simulink model "MavicProComplete"  (R2019a)
settings: Solver=VariableStepAuto  StartTime=0  StopTime=125  FixedStep=.01  RelTol=1e-3  EnableMultiTasking=on
InitFcn:
  | load('params/batteryModelSfun.mat');
  | load('params/DJI.mat');
  | load('params/DJIquadModel_X.mat');
  | load('params/motor.mat');
  | load('params/soc_ocv_new.mat');
model workspace (MAT data in the model file):
  Sig = Simulink.Signal
  Sig.DataType = 'auto'
  Sig.Dimensions = -1
  Sig.DimensionsMode = 'auto'
  Sig.Complexity = 'auto'
  Sig.SampleTime = -1
  Sig.SamplingMode = 'auto'
values from neighbouring files (symbols this model uses):
  P = block.ContStates.Data(1)    [quadcopterDynamicsSFunctionMod.m]
  Phi = block.ContStates.Data(4)    [quadcopterDynamicsSFunctionMod.m]
  Psi = block.ContStates.Data(6)    [quadcopterDynamicsSFunctionMod.m]
  Q = block.ContStates.Data(2)    [quadcopterDynamicsSFunctionMod.m]
  R = block.ContStates.Data(3)    [quadcopterDynamicsSFunctionMod.m]
  The = block.ContStates.Data(5)    [quadcopterDynamicsSFunctionMod.m]
  Z = block.ContStates.Data(12)    [quadcopterDynamicsSFunctionMod.m]
undefined symbols (not defined in the file or in its folder): Motor, quadModel
libraries: simulink x7
(part 1 of 2)
Description:
  | This is a configurable quadcopter simulation.
  | This Simulink model demonstates attitude control.
  | 
  | Additional quadcopter modeling and simulation materials available at:
  | github.com/dch33/Quad-Sim
  | 
  | Copyright (C) 2014 D. Hartman, K. Landis, S. Moreno, J. Kim, M. Mehrer
  | 
  | License:
  |     This program is free software: you can redistribute it and/or modify
  |     it under the terms of the GNU LESSER GENERAL PUBLIC LICENSE as published by
  |     the Free Software Foundation, either version 3 of the License, or
  |     (at your option) any later version.
  | 
  |     This program is distributed in the hope that it will be useful,
  |     but WITHOUT ANY WARRANTY; without even the implied warranty of
  |     MERCHANTABILITY or FITNESS FOR A PARTICULAR PURPOSE.  See the
  |     GNU General Public License for more details.
  | 
  |     You should have received a copy of the GNU LESSER GENERAL PUBLIC LICENSE
  |     along with this program.  If not, see <http://www.gnu.org/licenses/>.
settings Model: ModifiedComment=tdarrah -- Tue Jun 04 09:34:35 2019 -- Version 1.40  Creator=David Hartman  LastModifiedBy=tdarrah
settings Model: ModifiedHistory=|
  | tdarrah -- Tue Jun 04 09:34:35 2019 -- Version 1.40
  | 
  | tdarrah -- Tue Jun 04 05:29:55 2019 -- Version 1.39
  | 
  | tdarrah -- Mon Jun 03 18:31:35 2019 -- Version 1.38
  | closed the battery loop
  | 
  | tdarrah -- Mon Jun 03 18:20:30 2019 -- Version 1.37
  | added battery
  | 
  | 
  | tdarrah -- Mon Jun 03 17:58:08 2019 -- Version 1.36
  | incorporated our motors in model
  | 
  | 
  | Sahai Couso -- Fri May 10 11:35:12 2019 -- Version 1.35
  | 
  | Sahai Couso -- Fri May 10 10:41:34 2019 -- Version 1.34
  | 
  | Sahai Couso -- Fri May 10 10:40:52 2019 -- Version 1.33
  | 
  | Sahai Couso -- Fri May 10 10:30:50 2019 -- Version 1.32
  | 
  | Sahai Couso -- Fri May 10 10:24:25 2019 -- Version 1.31
  | 
  | Sahai Couso -- Wed May 08 22:16:35 2019 -- Version 1.30
  | 
  | Sahai Couso -- Wed May 08 22:15:23 2019 -- Version 1.29
  | 
  | Sahai Couso -- Wed May 08 22:14:58 2019 -- Version 1.28
  | 
  | Sahai Couso -- Wed May 08 22:04:36 2019 -- Version 1.27
  | 
  | Sahai Couso -- Wed May 08 22:04:16 2019 -- Version 1.26
  | 
  | Sahai Couso -- Wed May 08 21:57:14 2019 -- Version 1.25
  | 
  | Sahai Couso -- Wed May 08 21:54:04 2019 -- Version 1.24
  | 
  | Sahai Couso -- Wed May 08 21:53:17 2019 -- Version 1.23
  | 
  | Sahai Couso -- Wed May 08 21:48:07 2019 -- Version 1.22
  | 
  | Sahai Couso -- Wed May 08 21:35:53 2019 -- Version 1.21
  | 
  | Sahai Couso -- Wed May 08 21:28:21 2019 -- Version 1.19
  | 
  | Sahai Couso -- Wed May 08 21:28:21 2019 -- Version 1.19
  | 
  | Sahai Couso -- Wed May 08 21:25:30 2019 -- Version 1.18
  | 
  | Sahai Couso -- Wed May 08 21:23:06 2019 -- Version 1.17
  | 
  | Sahai Couso -- Wed May 08 13:57:34 2019 -- Version 1.16
  | 
  | Sahai Couso -- Wed May 08 00:58:43 2019 -- Version 1.15
  | 
  | Sahai Couso -- Wed May 08 00:58:03 2019 -- Version 1.14
  | 
  | Sahai Couso -- Tue May 07 23:55:58 2019 -- Version 1.13
  | 
  | Sahai Couso -- Tue May 07 23:08:00 2019 -- Version 1.12
  | 
  | Sahai Couso -- Tue May 07 23:06:52 2019 -- Version 1.11
  | 
  | Sahai Couso -- Tue May 07 22:57:09 2019 -- Version 1.10
  | 
  | Sahai Couso -- Tue May 07 22:48:57 2019 -- Version 1.9
  | 
  | Sahai Couso -- Tue May 07 21:40:08 2019 -- Version 1.8
  | 
  | Yves -- Tue Apr 04 13:12:37 2017 -- Version 1.7
  | 
  | Yves -- Tue Apr 04 13:10:33 2017 -- Version 1.6
  | 
  | davidhartman -- Fri Jun 06 23:19:51 2014 -- Version 1.5
  | 
  | 
  | davidhartman -- Fri Jun 06 22:53:10 2014 -- Version 1.3
settings SolverCC: AlgebraicLoopSolver=LineSearch  AutoInsertRateTranBlk=on
settings DataIOCC: SaveFormat=Array  SignalLogging=off  ReturnWorkspaceOutputs=off
settings OptimizationCC: DefaultParameterBehavior=Inlined  LifeSpan=inf
settings DebuggingCC: UnderspecifiedInitializationDetection=Classic  MergeDetectMultiDrivingBlocksExec=none  SolverPrmCheckMsg=warning  UniqueDataStoreMsg=warning  StateNameClashWarn=warning  PregeneratedLibrarySubsystemCodeDiagnostic=none  StrictBusMsg=WarnOnBusTreatedAsVector  SFUnexpectedBacktrackingDiag=warning  SFNoUnconditionalDefaultTransitionDiag=warning  SFExecutionAtInitializationDiag=none  ArithmeticOperatorsInVariantConditions=warning
settings HardwareCC: ProdBitPerPointer=32  ProdBitPerSizeT=32  ProdBitPerPtrDiffT=32  ProdLargestAtomicFloat=None  ProdIntDivRoundTo=Undefined  ProdEndianess=Unspecified  ProdWordSize=32  ProdHWDeviceType=32-bit Generic
settings ModelReferenceCC: PropagateSignalLabelsOutOfModel=off
settings SFSimCC: SimUseLocalCustomCode=off
settings RTWCC: RTWUseLocalCustomCode=off
settings CodeAppCC: StateflowObjectComments=on
settings GRTTargetCC: TargetLangStandard=C89/C90 (ANSI)  GeneratePreprocessorConditionals=Disable all
settings ConfigComp: CovMetricSettings=dw  CovHtmlReporting=on  CovSaveCumulativeToWorkspaceVar=on  CovSaveSingleToWorkspaceVar=on  CovExternalEMLEnable=off

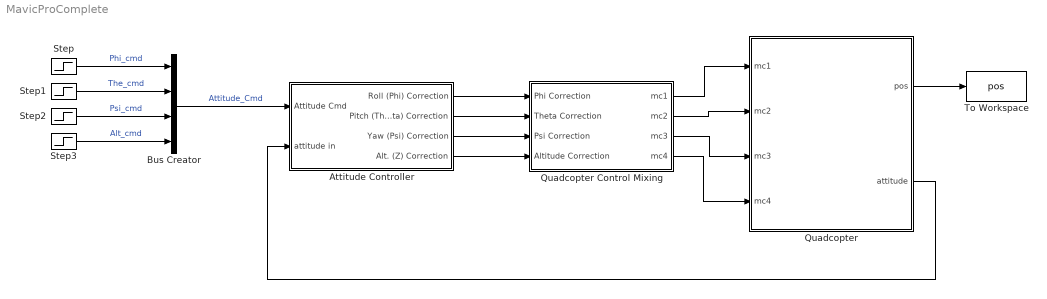
== system MavicProComplete ==
  Attitude Controller : Subsystem
  Bus Creator : BusCreator  Inputs=4
  Quadcopter : Subsystem
  Quadcopter Control Mixing : Subsystem
  Step : Step  Time=15  After=-.001  SampleTime=0
  Step1 : Step  Time=1000000  After=10*pi/180  SampleTime=0
  Step2 : Step  Time=1000000  After=45*pi/180  SampleTime=0
  Step3 : Step  Time=0  Before=10  After=10  SampleTime=0
  To Workspace : ToWorkspace  VariableName=pos  SampleTime=-1
      settings: Save2DSignal=2-D array (concatenate along first dimension)
  wires:
  Quadcopter/2(attitude) -> Attitude Controller/2(attitude in)
  Quadcopter Control Mixing/1(mc1) -> Quadcopter/1(mc1)
  Quadcopter Control Mixing/2(mc2) -> Quadcopter/2(mc2)
  Quadcopter Control Mixing/3(mc3) -> Quadcopter/3(mc3)
  Quadcopter Control Mixing/4(mc4) -> Quadcopter/4(mc4)
  Attitude Controller/1(Roll (Phi) Correction) -> Quadcopter Control Mixing/1(Phi Correction)
  Attitude Controller/2(Pitch (Theta) Correction) -> Quadcopter Control Mixing/2(Theta Correction)
  Attitude Controller/3(Yaw (Psi) Correction) -> Quadcopter Control Mixing/3(Psi Correction)
  Attitude Controller/4(Alt. (Z) Correction) -> Quadcopter Control Mixing/4(Altitude Correction)
  Step3/1 -> Bus Creator/4  "Alt_cmd"
  Step/1 -> Bus Creator/1  "Phi_cmd"
  Bus Creator/1 -> Attitude Controller/1(Attitude Cmd)  "Attitude_Cmd"
  Step2/1 -> Bus Creator/3  "Psi_cmd"
  Step1/1 -> Bus Creator/2  "The_cmd"
  Quadcopter/1(pos) -> To Workspace/1

== system MavicProComplete/Attitude Controller ==
  Attitude Cmd : Inport
  attitude in : Inport  Port=2
  Altitude (Z) Control : Subsystem  mask{Kpz=2, Kiz=1.1, Kdz=3.3, LimitOutput=on, USat=1, LSat=-1, GOffset=(sqrt((quadModel.mass*quadModel.g)/(4*quadModel.ct))-quadModel.b)/quadModel.cr}
      mask prompts: Kpz "Kp"; Kiz "Ki"; Kdz "Kd"; LimitOutput "Integral Saturation?"; USat "Upper saturation limit:"; LSat "Lower saturation limit:"; GOffset "Gravity Feedforward"
      mask help:
      | Adjust PID controller gains through this mask interface, or "look under mask" for more detailed adjustments.
      |
      | Note: Gravity Offset will not appear on block face as a value until simulation is run if it is the result of a formula involving the quadcopter model parameters.
      mask TypeOptions Kpz: Kpz/Gain
      mask TypeOptions Kiz: Kiz/Gain
      mask TypeOptions Kdz: Kdz/Gain
      mask TypeOptions LimitOutput:
      | Integrator
      | Limited/LimitOutput
      mask TypeOptions USat:
      | Integrator
      | Limited/UpperSaturationLimit
      mask TypeOptions LSat:
      | Integrator
      | Limited/LowerSaturationLimit
      mask TypeOptions GOffset: Gravity Offset (Level Flight)/Value
      mask Display:
      | fprintf(['Gravity Offset = ' num2str(GOffset) '\n' ...
      |     'Kp = ' num2str(Kpz) '\n' ...
      |     'Ki = ' num2str(Kiz) '\n' ...
      |     'Kd = ' num2str(Kdz) '\n' ...
      |     'Integral Saturation: ' LimitOutput]);
      | if strcmp(LimitOutput,'on')
      |     fprintf([' \n' ' \n' ' \n' ' \n' ' \n' '\n' ...
      |         'Limits: ' num2str(USat) ' to ' num2str(LSat)]);
      | end
  Bus Selector : BusSelector  OutputSignals=Phi,P,The,Q,Psi,R,Z
  Pitch (Theta) Control : Subsystem  mask{Kpt=2, Kit=1.1, Kdt=1.2, LimitOutput=on, USat=1, LSat=-1}
      mask prompts: Kpt "Kp"; Kit "Ki"; Kdt "Kd"; LimitOutput "Integral Saturation?"; USat "Upper saturation limit:"; LSat "Lower saturation limit:"
      mask help: Adjust PID controller gains through this mask interface, or "look under mask" for more detailed adjustments.
      mask TypeOptions Kpt: Kpt/Gain
      mask TypeOptions Kit: Kit/Gain
      mask TypeOptions Kdt: Kdt/Gain
      mask TypeOptions LimitOutput:
      | Integrator
      | Limited/LimitOutput
      mask TypeOptions USat:
      | Integrator
      | Limited/UpperSaturationLimit
      mask TypeOptions LSat:
      | Integrator
      | Limited/LowerSaturationLimit
      mask Display:
      | fprintf(['Kp = ' num2str(Kpt) '\n' ...
      |     'Ki = ' num2str(Kit) '\n' ...
      |     'Kd = ' num2str(Kdt) '\n' ...
      |     'Integral Saturation: ' LimitOutput]);
      | if strcmp(LimitOutput,'on')
      |     fprintf([' \n' ' \n' ' \n' ' \n' '\n' ...
      |         'Limits: ' num2str(USat) ' to ' num2str(LSat)]);
      | end
  "Roll (Phi) Control " : Subsystem  mask{Kpp=2.0, Kip=1.1, Kdp=1.2, LimitOutput=on, USat=1, LSat=-1}
      mask prompts: Kpp "Kp"; Kip "Ki"; Kdp "Kd"; LimitOutput "Integral Saturation:"; USat "Upper saturation limit:"; LSat "Lower saturation limit:"
      mask help:
      | Adjust PID controller gains through this mask interface, or "look under mask"
      | for more detailed adjustments.
      mask TypeOptions Kpp: Kpp/Gain
      mask TypeOptions Kip: Kip/Gain
      mask TypeOptions Kdp: Kdp/Gain
      mask TypeOptions LimitOutput:
      | Integrator
      | Limited/LimitOutput
      mask TypeOptions USat:
      | Integrator
      | Limited/UpperSaturationLimit
      mask TypeOptions LSat:
      | Integrator
      | Limited/LowerSaturationLimit
      mask Display:
      | fprintf(['Kp = ' num2str(Kpp) '\n' ...
      |     'Ki = ' num2str(Kip) '\n' ...
      |     'Kd = ' num2str(Kdp) '\n'...
      |     'Integral Saturation: ' LimitOutput]);
      | if strcmp(LimitOutput,'on')
      |     fprintf([' \n' ' \n' ' \n' ' \n' '\n' ...
      |         'Limits: ' num2str(USat) ' to ' num2str(LSat)]);
      | end
  Yaw (Psi) Control : Subsystem  mask{Kps=4, Kis=0.5, Kds=3.5, LimitOutput=on, USat=1, LSat=-1}
      mask prompts: Kps "Kp"; Kis "Ki"; Kds "Kd"; LimitOutput "Integral Saturation?"; USat "Upper saturation limit:"; LSat "Lower saturation limit:"
      mask help: Adjust PID controller gains through this mask interface, or "look under mask" for more detailed adjustments.
      mask TypeOptions Kps: Kps/Gain
      mask TypeOptions Kis: Kit/Gain
      mask TypeOptions Kds: Kds/Gain
      mask TypeOptions LimitOutput:
      | Integrator
      | Limited/LimitOutput
      mask TypeOptions USat:
      | Integrator
      | Limited/UpperSaturationLimit
      mask TypeOptions LSat:
      | Integrator
      | Limited/LowerSaturationLimit
      mask Display:
      | fprintf(['Kp = ' num2str(Kps) '\n' ...
      |     'Ki = ' num2str(Kis) '\n' ...
      |     'Kd = ' num2str(Kds) '\n' ...
      |     'Integral Saturation: ' LimitOutput]);
      | if strcmp(LimitOutput,'on')
      |     fprintf([' \n' ' \n' ' \n' ' \n' '\n' ...
      |         'Limits: ' num2str(USat) ' to ' num2str(LSat)]);
      | end
  Roll (Phi) Correction : Outport
  Pitch (Theta) Correction : Outport  Port=2
  Yaw (Psi) Correction : Outport  Port=3
  Alt. (Z) Correction : Outport  Port=4
  wires:
  Bus Selector/6 -> Yaw (Psi) Control/3(R State)  "<R>"
  Bus Selector/4 -> Pitch (Theta) Control/3(Q State)  "<Q>"
  Bus Selector/2 -> "Roll (Phi) Control "/3(P)  "<P>"
  Bus Selector/3 -> Pitch (Theta) Control/2(Theta State)  "<The>"
  Attitude Cmd/1 -> "Roll (Phi) Control "/1("Attitude Command "), Pitch (Theta) Control/1(Attitude Command), Yaw (Psi) Control/1(Attitude Command), Altitude (Z) Control/1(Desired Z)
  Bus Selector/7 -> Altitude (Z) Control/2(Z State)  "<Z>"
  Altitude (Z) Control/1(Alt. (Z) Correction) -> Alt. (Z) Correction/1
  Bus Selector/5 -> Yaw (Psi) Control/2(Psi State)  "<Psi>"
  Yaw (Psi) Control/1(Psi Correction) -> Yaw (Psi) Correction/1
  Pitch (Theta) Control/1(Theta Correction) -> Pitch (Theta) Correction/1
  attitude in/1 -> Bus Selector/1
  Bus Selector/1 -> "Roll (Phi) Control "/2(Phi State)  "<Phi>"
  "Roll (Phi) Control "/1(Phi Correction) -> Roll (Phi) Correction/1

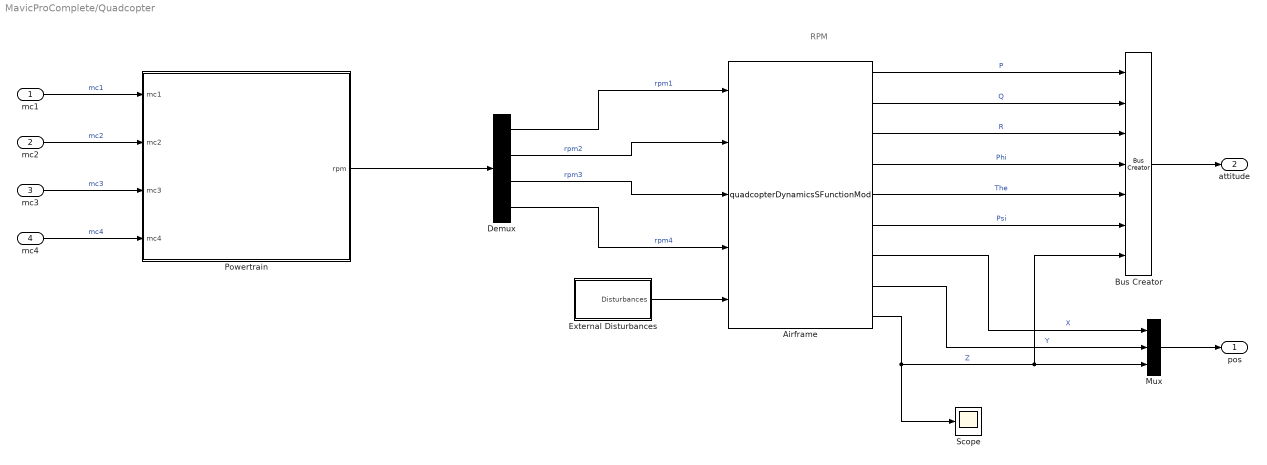
== system MavicProComplete/Quadcopter ==
  note: RPM
  mc1 : Inport
  mc2 : Inport  Port=2
  mc3 : Inport  Port=3
  mc4 : Inport  Port=4
  Airframe : M-S-Function  FunctionName=quadcopterDynamicsSFunctionMod  Parameters=quadModel, IC
      mask Display:
      | port_label('input', 1, 'RPM1')
      | port_label('input', 2, 'RPM2')
      | port_label('input', 3, 'RPM3')
      | port_label('input', 4, 'RPM4')
      | port_label('input', 5, 'Disturbances')
      | port_label('output', 1, 'P')
      | port_label('output', 2, 'Q')
      | port_label('output', 3, 'R')
      | port_label('output', 4, 'Phi')
      | port_label('output', 5, 'The')
      | port_label('output', 6, 'Psi')
      | port_label('output', 7, 'X')
      | port_label('output', 8, 'Y')
      | port_label('output', 9, 'Z')
  Bus Creator : BusCreator  Inputs=P,Q,R,Phi,The,Psi,Z
  Demux : Demux
  External Disturbances : Subsystem
  Mux : Mux  Inputs=3
  Powertrain : Subsystem
  Scope : Scope
  pos : Outport
  attitude : Outport  Port=2
  wires:
  External Disturbances/1("Disturbances ") -> Airframe/5
  Bus Creator/1 -> attitude/1
  Airframe/9 -> Scope/1, Bus Creator/7, Mux/3  "Z"
  Airframe/8 -> Mux/2  "Y"
  Airframe/7 -> Mux/1  "X"
  Airframe/6 -> Bus Creator/6  "Psi"
  Airframe/5 -> Bus Creator/5  "The"
  Airframe/4 -> Bus Creator/4  "Phi"
  Airframe/3 -> Bus Creator/3  "R"
  Airframe/2 -> Bus Creator/2  "Q"
  Airframe/1 -> Bus Creator/1  "P"
  Mux/1 -> pos/1
  Demux/1 -> Airframe/1  "rpm1"
  Demux/2 -> Airframe/2  "rpm2"
  Demux/3 -> Airframe/3  "rpm3"
  Demux/4 -> Airframe/4  "rpm4"
  mc1/1 -> Powertrain/1(mc1)  "mc1"
  mc2/1 -> Powertrain/2(mc2)  "mc2"
  mc3/1 -> Powertrain/3(mc3)  "mc3"
  mc4/1 -> Powertrain/4(mc4)  "mc4"
  Powertrain/1(rpm) -> Demux/1

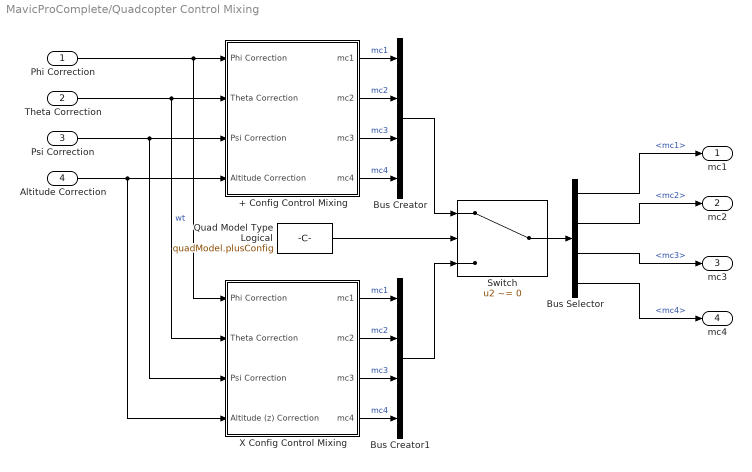
== system MavicProComplete/Quadcopter Control Mixing ==
  Phi Correction : Inport
  Theta Correction : Inport  Port=2
  Psi Correction : Inport  Port=3
  Altitude Correction : Inport  Port=4
  + Config Control Mixing : Subsystem
  Bus Creator : BusCreator  Inputs=4
  Bus Creator1 : BusCreator  Inputs=4
  Bus Selector : BusSelector  OutputSignals=mc1,mc2,mc3,mc4
  Quad Model Type Logical : Constant  Value=quadModel.plusConfig
  Switch : Switch  Criteria=u2 ~= 0
  X Config Control Mixing : Subsystem
  mc1 : Outport
  mc2 : Outport  Port=2
  mc3 : Outport  Port=3
  mc4 : Outport  Port=4
  wires:
  Switch/1 -> Bus Selector/1
  Quad Model Type Logical/1 -> Switch/2
  Bus Selector/4 -> mc4/1  "<mc4>"
  Bus Selector/3 -> mc3/1  "<mc3>"
  Bus Selector/2 -> mc2/1  "<mc2>"
  Bus Selector/1 -> mc1/1  "<mc1>"
  Bus Creator1/1 -> Switch/3
  X Config Control Mixing/4(mc4) -> Bus Creator1/4  "mc4"
  X Config Control Mixing/3(mc3) -> Bus Creator1/3  "mc3"
  X Config Control Mixing/2(mc2) -> Bus Creator1/2  "mc2"
  X Config Control Mixing/1(mc1) -> Bus Creator1/1  "mc1"
  Bus Creator/1 -> Switch/1
  + Config Control Mixing/4(mc4) -> Bus Creator/4  "mc4"
  + Config Control Mixing/3(mc3) -> Bus Creator/3  "mc3"
  + Config Control Mixing/2(mc2) -> Bus Creator/2  "mc2"
  + Config Control Mixing/1(mc1) -> Bus Creator/1  "mc1"
  Altitude Correction/1 -> + Config Control Mixing/4(Altitude Correction), X Config Control Mixing/4(Altitude (z) Correction)
  Psi Correction/1 -> + Config Control Mixing/3(Psi Correction), X Config Control Mixing/3(Psi Correction)
  Theta Correction/1 -> + Config Control Mixing/2(Theta Correction), X Config Control Mixing/2(Theta Correction)  "wt"
  Phi Correction/1 -> + Config Control Mixing/1(Phi Correction), X Config Control Mixing/1(Phi Correction)

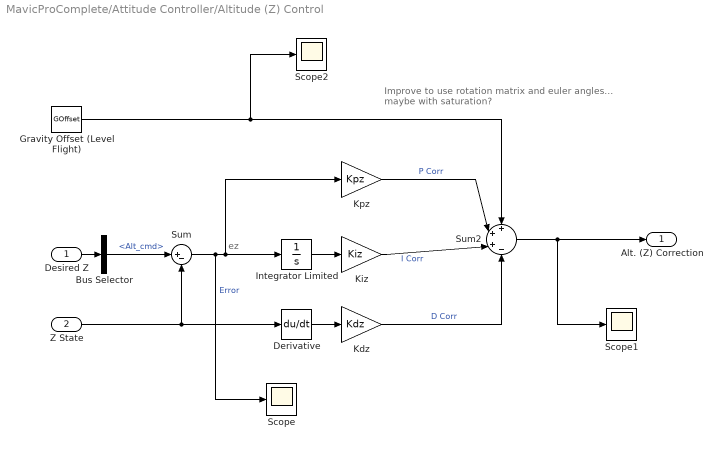
== system MavicProComplete/Attitude Controller/Altitude (Z) Control ==
  note: ez
  note: Improve to use rotation matrix and euler angles...
      | maybe with saturation?
  Desired Z : Inport
  Z State : Inport  Port=2
  Bus Selector : BusSelector  OutputSignals=Alt_cmd
  Derivative : Derivative
  Gravity Offset (Level Flight) : Constant  Value=GOffset
  Integrator Limited : Integrator  LimitOutput=on  UpperSaturationLimit=USat  LowerSaturationLimit=LSat
  Kdz : Gain  Gain=Kdz
  Kiz : Gain  Gain=Kiz
  Kpz : Gain  Gain=Kpz
  Scope : Scope
  Scope1 : Scope
  Scope2 : Scope
  Sum : Sum  Inputs=|+-
  Sum2 : Sum  Inputs=+++-
  Alt. (Z) Correction : Outport
  wires:
  Derivative/1 -> Kdz/1
  Bus Selector/1 -> Sum/1  "<Alt_cmd>"
  Integrator Limited/1 -> Kiz/1
  Kdz/1 -> Sum2/4  "D Corr"
  Kiz/1 -> Sum2/3  "I Corr"
  Sum/1 -> Scope/1, Kpz/1, Integrator Limited/1  "Error"
  Kpz/1 -> Sum2/2  "P Corr"
  Sum2/1 -> Scope1/1, Alt. (Z) Correction/1
  Z State/1 -> Sum/2, Derivative/1
  Desired Z/1 -> Bus Selector/1
  Gravity Offset (Level Flight)/1 -> Scope2/1, Sum2/1

== system MavicProComplete/Attitude Controller/Pitch (Theta) Control ==
  Attitude Command : Inport
  Theta State : Inport  Port=2
  Q State : Inport  Port=3
  Bus Selector : BusSelector  OutputSignals=The_cmd
  Integrator Limited : Integrator  LimitOutput=on  UpperSaturationLimit=USat  LowerSaturationLimit=LSat
  Kdt : Gain  Gain=Kdt
  Kit : Gain  Gain=Kit
  Kpt : Gain  Gain=Kpt
  Sum : Sum  Inputs=|+-
  Sum1 : Sum  Inputs=++-
  Theta Correction : Outport
  wires:
  Q State/1 -> Kdt/1
  Bus Selector/1 -> Sum/1  "<The_cmd>"
  Integrator Limited/1 -> Kit/1
  Kit/1 -> Sum1/2  "I Corr"
  Kdt/1 -> Sum1/3  "D Corr"
  Kpt/1 -> Sum1/1  "P Corr"
  Sum1/1 -> Theta Correction/1
  Theta State/1 -> Sum/2
  Attitude Command/1 -> Bus Selector/1
  Sum/1 -> Kpt/1, Integrator Limited/1  "Error"

== system MavicProComplete/Attitude Controller/Roll (Phi) Control  ==
  "Attitude Command " : Inport
  Phi State : Inport  Port=2
  P : Inport  Port=3
  Bus Selector : BusSelector  OutputSignals=Phi_cmd
  Integrator Limited : Integrator  LimitOutput=on  UpperSaturationLimit=USat  LowerSaturationLimit=LSat
  Kdp : Gain  Gain=Kdp
  Kip : Gain  Gain=Kip
  Kpp : Gain  Gain=Kpp
  Sum : Sum  Inputs=|+-
  Sum1 : Sum  Inputs=++-
  Phi Correction : Outport
  wires:
  P/1 -> Kdp/1
  Bus Selector/1 -> Sum/1  "<Phi_cmd>"
  "Attitude Command "/1 -> Bus Selector/1
  Integrator Limited/1 -> Kip/1
  Kip/1 -> Sum1/2  "I Corr"
  Kdp/1 -> Sum1/3  "D Corr"
  Kpp/1 -> Sum1/1  "P Corr"
  Sum1/1 -> Phi Correction/1
  Phi State/1 -> Sum/2
  Sum/1 -> Kpp/1, Integrator Limited/1  "Error"

== system MavicProComplete/Attitude Controller/Yaw (Psi) Control ==
  Attitude Command : Inport
  Psi State : Inport  Port=2
  R State : Inport  Port=3
  Bus Selector : BusSelector  OutputSignals=Psi_cmd
  Integrator Limited : Integrator  LimitOutput=on  UpperSaturationLimit=USat  LowerSaturationLimit=LSat
  Kds : Gain  Gain=Kds
  Kit : Gain  Gain=Kis
  Kps : Gain  Gain=Kps
  Sum : Sum  Inputs=|+-
  Sum1 : Sum  Inputs=++-
  Psi Correction : Outport
  wires:
  R State/1 -> Kds/1
  Bus Selector/1 -> Sum/1  "<Psi_cmd>"
  Integrator Limited/1 -> Kit/1
  Kit/1 -> Sum1/2  "I Corr"
  Kds/1 -> Sum1/3  "D Corr"
  Kps/1 -> Sum1/1  "P Corr"
  Psi State/1 -> Sum/2
  Sum1/1 -> Psi Correction/1
  Attitude Command/1 -> Bus Selector/1
  Sum/1 -> Kps/1, Integrator Limited/1  "Error"

== system MavicProComplete/Quadcopter/External Disturbances ==
  note: Note: Torques are in units of N*m, Forces in N
      | Torques are applied to the BODY coordinate system.
      | Forces are applied from the WORLD coordinate system!
      | This can be changed by adjusting the equations within the S-function.
  Bus Creator : BusCreator  Inputs=6
  Bus to Vector : BusToVector
  Constant{2..6} (5 alike) : Constant  Value=0
  Step : Step  After=0  SampleTime=0
  "Disturbances " : Outport
  wires:
  Constant5/1 -> Bus Creator/6  "Force_z-axis"
  Constant4/1 -> Bus Creator/5  "Force_y-axis"
  Constant3/1 -> Bus Creator/4  "Force_x-axis"
  Constant2/1 -> Bus Creator/3  "Tau_bz-axis"
  Step/1 -> Bus Creator/2  "Tau_by-axis"
  Constant6/1 -> Bus Creator/1  "Tau_bx-axis"
  Bus Creator/1 -> Bus to Vector/1
  Bus to Vector/1 -> "Disturbances "/1

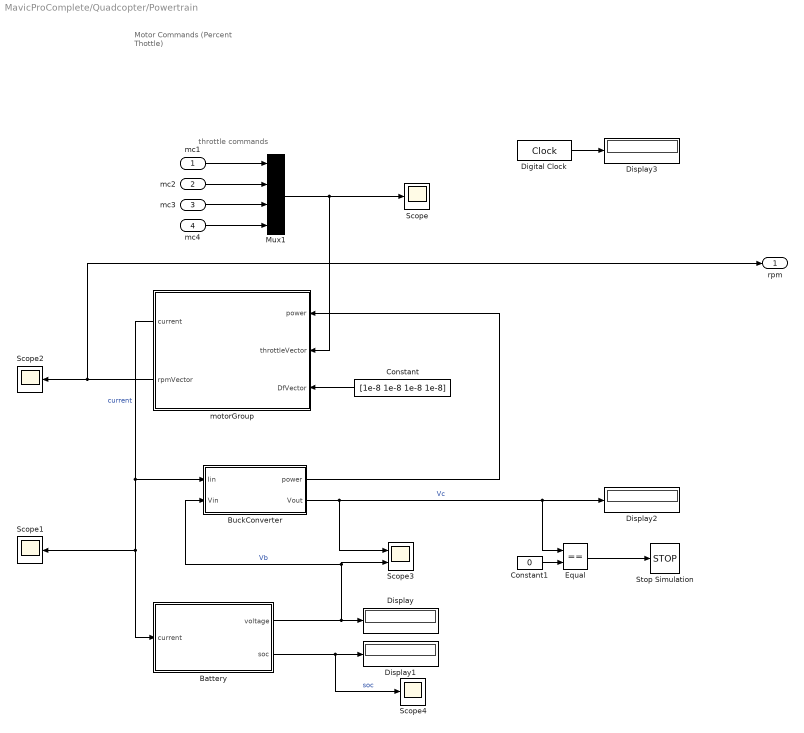
== system MavicProComplete/Quadcopter/Powertrain ==
  note: throttle commands
  note: Motor Commands
      | (Percent Thottle)
  mc1 : Inport
  mc2 : Inport  Port=2
  mc3 : Inport  Port=3
  mc4 : Inport  Port=4
  Battery : Subsystem
  BuckConverter : Subsystem
  Constant : Constant  Value=[1e-8 1e-8 1e-8 1e-8]
  Constant1 : Constant  Value=0
  Digital Clock : DigitalClock
      mask Display: disp('Sim Time');
  Display{,1..3} (4 alike) : Display
  Equal : RelationalOperator  Operator===  OutDataTypeStr=boolean  RndMeth=Simplest
  Mux1 : Mux
  Scope{,1..2,4} (4 alike) : Scope
  Scope3 : Scope  NumInputPorts=2
  Stop Simulation : Stop
  motorGroup : Subsystem
  rpm : Outport
  wires:
  Constant1/1 -> Equal/2
  Constant/1 -> motorGroup/3(DfVector)
  mc3/1 -> Mux1/3
  motorGroup/2(rpmVector) -> rpm/1, Scope2/1
  Digital Clock/1 -> Display3/1
  mc1/1 -> Mux1/1
  mc4/1 -> Mux1/4
  BuckConverter/2(Vout) -> Scope3/1, Equal/1, Display2/1  "Vc"
  Battery/2(soc) -> Scope4/1, Display1/1  "soc"
  Mux1/1 -> motorGroup/2(throttleVector), Scope/1
  Equal/1 -> Stop Simulation/1
  Battery/1(voltage) -> BuckConverter/2(Vin), Scope3/2, Display/1  "Vb"
  BuckConverter/1(power) -> motorGroup/1(power)
  mc2/1 -> Mux1/2
  motorGroup/1(current) -> BuckConverter/1(Iin), Battery/1(current), Scope1/1  "current"

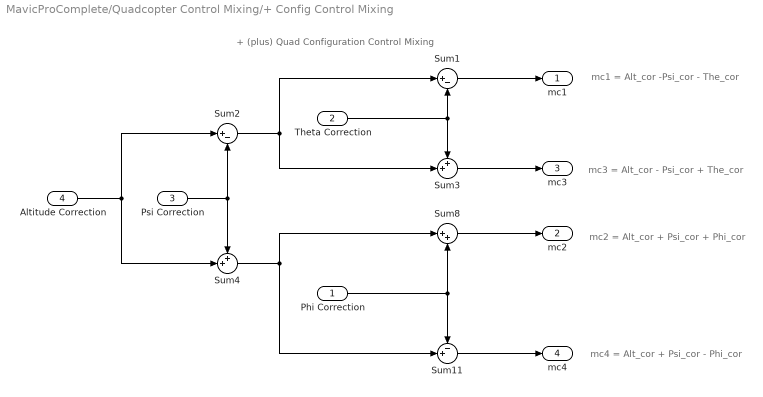
== system MavicProComplete/Quadcopter Control Mixing/+ Config Control Mixing ==
  note: mc1 = Alt_cor -Psi_cor - The_cor
  note: mc3 = Alt_cor - Psi_cor + The_cor
  note: mc4 = Alt_cor + Psi_cor - Phi_cor
  note: + (plus) Quad Configuration Control Mixing
  note: mc2 = Alt_cor + Psi_cor + Phi_cor
  Phi Correction : Inport
  Theta Correction : Inport  Port=2
  Psi Correction : Inport  Port=3
  Altitude Correction : Inport  Port=4
  Sum1 : Sum  Inputs=|+-
  Sum11 : Sum  Inputs=-+|
  Sum2 : Sum  Inputs=|+-
  Sum3 : Sum  Inputs=++|
  Sum4 : Sum  Inputs=++|
  Sum8 : Sum  Inputs=|++
  mc1 : Outport
  mc2 : Outport  Port=2
  mc3 : Outport  Port=3
  mc4 : Outport  Port=4
  wires:
  Sum11/1 -> mc4/1
  Sum8/1 -> mc2/1
  Sum3/1 -> mc3/1
  Sum1/1 -> mc1/1
  Phi Correction/1 -> Sum11/1, Sum8/2
  Sum4/1 -> Sum8/1, Sum11/2
  Psi Correction/1 -> Sum2/2, Sum4/1
  Sum2/1 -> Sum1/1, Sum3/2
  Altitude Correction/1 -> Sum4/2, Sum2/1
  Theta Correction/1 -> Sum3/1, Sum1/2

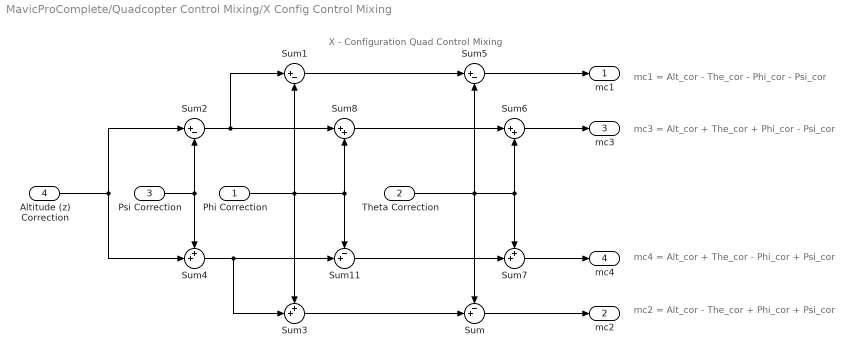
== system MavicProComplete/Quadcopter Control Mixing/X Config Control Mixing ==
  note: mc4 = Alt_cor + The_cor - Phi_cor + Psi_cor
  note: mc2 = Alt_cor - The_cor + Phi_cor + Psi_cor
  note: mc3 = Alt_cor + The_cor + Phi_cor - Psi_cor
  note: X - Configuration Quad Control Mixing
  note: mc1 = Alt_cor - The_cor - Phi_cor - Psi_cor
  Phi Correction : Inport
  Theta Correction : Inport  Port=2
  Psi Correction : Inport  Port=3
  Altitude (z) Correction : Inport  Port=4
  Sum : Sum  Inputs=-+|
  Sum1 : Sum  Inputs=|+-
  Sum11 : Sum  Inputs=-+|
  Sum2 : Sum  Inputs=|+-
  Sum3 : Sum  Inputs=++|
  Sum4 : Sum  Inputs=++|
  Sum5 : Sum  Inputs=|+-
  Sum6 : Sum  Inputs=|++
  Sum7 : Sum  Inputs=++|
  Sum8 : Sum  Inputs=|++
  mc1 : Outport
  mc2 : Outport  Port=2
  mc3 : Outport  Port=3
  mc4 : Outport  Port=4
  wires:
  Sum/1 -> mc2/1
  Altitude (z) Correction/1 -> Sum4/2, Sum2/1
  Sum7/1 -> mc4/1
  Sum6/1 -> mc3/1
  Sum5/1 -> mc1/1
  Sum11/1 -> Sum7/2
  Sum8/1 -> Sum6/1
  Sum1/1 -> Sum5/1
  Theta Correction/1 -> Sum/1, Sum5/2, Sum6/2, Sum7/1
  Sum3/1 -> Sum/2
  Sum4/1 -> Sum11/2, Sum3/2
  Phi Correction/1 -> Sum11/1, Sum8/2, Sum1/2, Sum3/1
  Psi Correction/1 -> Sum2/2, Sum4/1
  Sum2/1 -> Sum1/1, Sum8/1

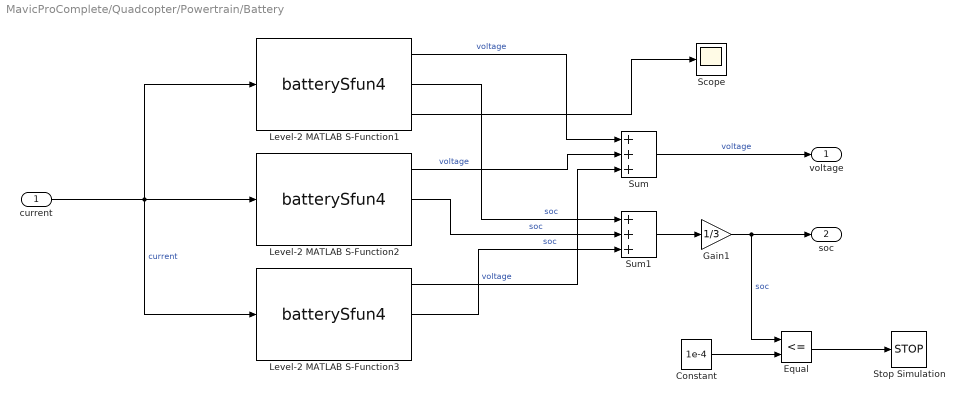
== system MavicProComplete/Quadcopter/Powertrain/Battery ==
  current : Inport
  Constant : Constant  Value=1e-4
  Equal : RelationalOperator  Operator=<=  OutDataTypeStr=boolean  RndMeth=Simplest
  Gain1 : Gain  Gain=1/3
  Level-2 MATLAB S-Function1 : M-S-Function  FunctionName=batterySfun4  Parameters=battery, soc_ocv, .001
      mask Display:
      | port_label('input', 1, 'current');
      | port_label('output', 1, 'voltage');
      | port_label('output', 2, 'soc');
  Level-2 MATLAB S-Function2 : M-S-Function  FunctionName=batterySfun4  Parameters=battery, soc_ocv, .001
      mask Display:
      | port_label('input', 1, 'current');
      | port_label('output', 1, 'voltage');
      | port_label('output', 2, 'soc');
  Level-2 MATLAB S-Function3 : M-S-Function  FunctionName=batterySfun4  Parameters=battery, soc_ocv, .001
      mask Display:
      | port_label('input', 1, 'current');
      | port_label('output', 1, 'voltage');
      | port_label('output', 2, 'soc');
  Scope : Scope
  Stop Simulation : Stop
  Sum : Sum  Inputs=+++
  Sum1 : Sum  Inputs=+++
  voltage : Outport
  soc : Outport  Port=2
  wires:
  Level-2 MATLAB S-Function2/1 -> Sum/2  "voltage"
  Level-2 MATLAB S-Function1/1 -> Sum/1  "voltage"
  Level-2 MATLAB S-Function2/2 -> Sum1/2  "soc"
  Sum1/1 -> Gain1/1
  Gain1/1 -> Equal/1, soc/1  "soc"
  Level-2 MATLAB S-Function1/2 -> Sum1/1  "soc"
  Level-2 MATLAB S-Function3/2 -> Sum1/3  "soc"
  current/1 -> Level-2 MATLAB S-Function3/1, Level-2 MATLAB S-Function1/1, Level-2 MATLAB S-Function2/1  "current"
  Level-2 MATLAB S-Function3/1 -> Sum/3  "voltage"
  Sum/1 -> voltage/1  "voltage"
  Level-2 MATLAB S-Function1/3 -> Scope/1
  Constant/1 -> Equal/2
  Equal/1 -> Stop Simulation/1

== system MavicProComplete/Quadcopter/Powertrain/BuckConverter ==
  Iin : Inport
  Vin : Inport  Port=2
  Constant : Constant  Value=0
  Constant2 : Constant  Value=11.4
  If : If  IfExpression=u1 > 10.5
  If Action Subsystem : Subsystem  TreatAsAtomicUnit=on
  If Action Subsystem1 : Subsystem  TreatAsAtomicUnit=on
  Product : Product
  Switch : Switch  Criteria=u2 > Threshold  Threshold=10.5
  power : Outport
  Vout : Outport  Port=2
  wires:
  Product/1 -> power/1
  Iin/1 -> Product/1
  If/1 -> If Action Subsystem/Action
  If/2 -> If Action Subsystem1/Action
  Constant/1 -> If Action Subsystem1/1(In1)
  If Action Subsystem/1(Out1) -> Switch/1
  If Action Subsystem1/1(Out1) -> Switch/3
  Constant2/1 -> If Action Subsystem/1(In1)
  Vin/1 -> Switch/2, If/1
  Switch/1 -> Product/2, Vout/1

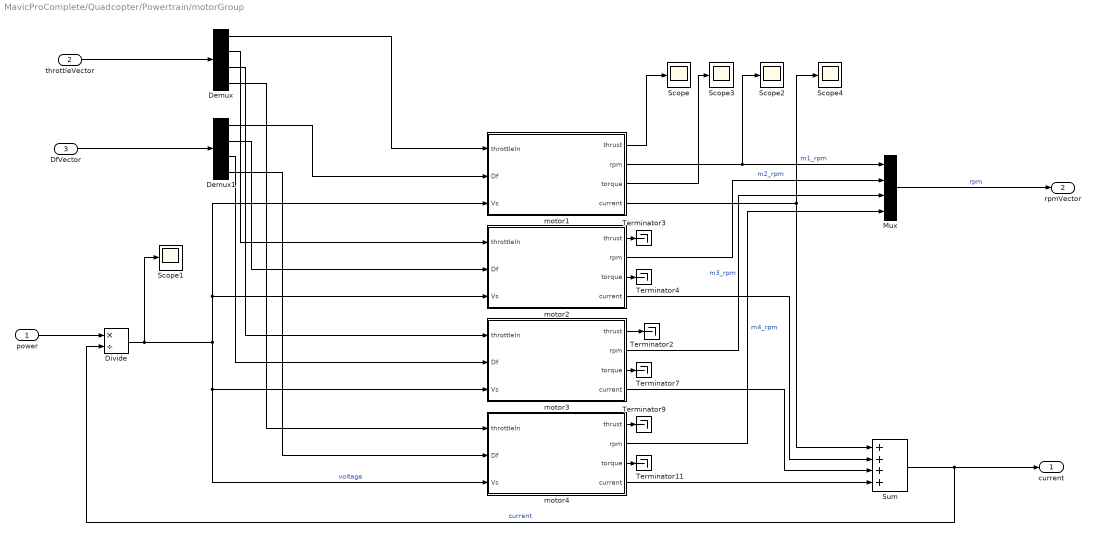
== system MavicProComplete/Quadcopter/Powertrain/motorGroup ==
  power : Inport
  throttleVector : Inport  Port=2  PortDimensions=4
  DfVector : Inport  Port=3  PortDimensions=4
  Demux : Demux
  Demux1 : Demux
  Divide : Product  Inputs=*/
  Mux : Mux
  Scope{,1..4} (5 alike) : Scope
  Sum : Sum  Inputs=++++
  Terminator{2..4,7,9,11} (6 alike) : Terminator
  motor1 : Subsystem
  motor2 : Subsystem
  motor3 : Subsystem
  motor4 : Subsystem
  current : Outport
  rpmVector : Outport  Port=2
  wires:
  Demux1/2 -> motor2/2(Df)
  Demux1/4 -> motor4/2(Df)
  Divide/1 -> Scope1/1, motor1/3(Vs), motor2/3(Vs), motor4/3(Vs), motor3/3(Vs)  "voltage"
  Demux1/1 -> motor1/2(Df)
  Sum/1 -> current/1, Divide/2  "current"
  Demux1/3 -> motor3/2(Df)
  motor1/4(current) -> Scope4/1, Sum/1
  power/1 -> Divide/1
  Demux/4 -> motor4/1(throttleIn)
  Demux/3 -> motor3/1(throttleIn)
  Demux/2 -> motor2/1(throttleIn)
  Demux/1 -> motor1/1(throttleIn)
  throttleVector/1 -> Demux/1
  DfVector/1 -> Demux1/1
  motor4/4(current) -> Sum/4
  motor3/4(current) -> Sum/3
  motor2/4(current) -> Sum/2
  motor4/2(rpm) -> Mux/4  "m4_rpm"
  motor3/2(rpm) -> Mux/3  "m3_rpm"
  motor2/2(rpm) -> Mux/2  "m2_rpm"
  motor1/2(rpm) -> Scope2/1, Mux/1  "m1_rpm"
  Mux/1 -> rpmVector/1  "rpm"
  motor1/1(thrust) -> Scope/1
  motor4/3(torque) -> Terminator11/1
  motor1/3(torque) -> Scope3/1
  motor2/3(torque) -> Terminator4/1
  motor3/3(torque) -> Terminator7/1
  motor4/1(thrust) -> Terminator9/1
  motor3/1(thrust) -> Terminator2/1
  motor2/1(thrust) -> Terminator3/1

== system MavicProComplete/Quadcopter/Powertrain/BuckConverter/If Action Subsystem ==
  In1 : Inport
  Action Port : ActionPort  ActionPortLabel=if(u1 > 10.5)
  Out1 : Outport
  wires:
  In1/1 -> Out1/1

== system MavicProComplete/Quadcopter/Powertrain/BuckConverter/If Action Subsystem1 ==
  In1 : Inport
  Action Port : ActionPort  ActionPortLabel=else
  Out1 : Outport
  wires:
  In1/1 -> Out1/1

== system MavicProComplete/Quadcopter/Powertrain/motorGroup/motor1 ==
  note: Throttle cutoff can simulate the fact that the motor doesn't
      | spin until a minimum throttle point is reached. This introduces
      | a jump discontinuity in low throttle performance.
  note: These saturations model a SIGNAL LIMITATION.
      | Other intentional control saturations might be introduced in the
      | control loop to achieve better stability and consistency.
  throttleIn : Inport
  Df : Inport  Port=2
  Vs : Inport  Port=3
  Scope : Scope
  Signal_Saturation_4 : Saturate  UpperLimit=100  LowerLimit=0
  Throttle To RPM Gain and Cutoff_8 : Subsystem
  motorRotor4 : Subsystem
  thrust : Outport
  rpm : Outport  Port=2
  torque : Outport  Port=3
  current : Outport  Port=4
  wires:
  Throttle To RPM Gain and Cutoff_8/1(Out5) -> motorRotor4/1(V), Scope/1
  motorRotor4/4(current) -> current/1
  motorRotor4/2(rpm) -> rpm/1
  throttleIn/1 -> Signal_Saturation_4/1
  motorRotor4/3(torque) -> torque/1
  motorRotor4/1(thrust) -> thrust/1
  Signal_Saturation_4/1 -> Throttle To RPM Gain and Cutoff_8/1(In5)
  Df/1 -> motorRotor4/2(Df)
  Vs/1 -> Throttle To RPM Gain and Cutoff_8/2(Vs)

== system MavicProComplete/Quadcopter/Powertrain/motorGroup/motor2 ==
  note: Throttle cutoff can simulate the fact that the motor doesn't
      | spin until a minimum throttle point is reached. This introduces
      | a jump discontinuity in low throttle performance.
  note: These saturations model a SIGNAL LIMITATION.
      | Other intentional control saturations might be introduced in the
      | control loop to achieve better stability and consistency.
  throttleIn : Inport
  Df : Inport  Port=2
  Vs : Inport  Port=3
  Scope : Scope
  Signal_Saturation_4 : Saturate  UpperLimit=100  LowerLimit=0
  Throttle To RPM Gain and Cutoff_8 : Subsystem
  motorRotor4 : Subsystem
  thrust : Outport
  rpm : Outport  Port=2
  torque : Outport  Port=3
  current : Outport  Port=4
  wires:
  Throttle To RPM Gain and Cutoff_8/1(Out5) -> motorRotor4/1(V), Scope/1
  motorRotor4/4(current) -> current/1
  motorRotor4/2(rpm) -> rpm/1
  throttleIn/1 -> Signal_Saturation_4/1
  motorRotor4/3(torque) -> torque/1
  motorRotor4/1(thrust) -> thrust/1
  Signal_Saturation_4/1 -> Throttle To RPM Gain and Cutoff_8/1(In5)
  Df/1 -> motorRotor4/2(Df)
  Vs/1 -> Throttle To RPM Gain and Cutoff_8/2(Vs)

== system MavicProComplete/Quadcopter/Powertrain/motorGroup/motor3 ==
  note: Throttle cutoff can simulate the fact that the motor doesn't
      | spin until a minimum throttle point is reached. This introduces
      | a jump discontinuity in low throttle performance.
  note: These saturations model a SIGNAL LIMITATION.
      | Other intentional control saturations might be introduced in the
      | control loop to achieve better stability and consistency.
  throttleIn : Inport
  Df : Inport  Port=2
  Vs : Inport  Port=3
  Scope : Scope
  Signal_Saturation_4 : Saturate  UpperLimit=100  LowerLimit=0
  Throttle To RPM Gain and Cutoff_8 : Subsystem
  motorRotor4 : Subsystem
  thrust : Outport
  rpm : Outport  Port=2
  torque : Outport  Port=3
  current : Outport  Port=4
  wires:
  Throttle To RPM Gain and Cutoff_8/1(Out5) -> motorRotor4/1(V), Scope/1
  motorRotor4/4(current) -> current/1
  motorRotor4/2(rpm) -> rpm/1
  throttleIn/1 -> Signal_Saturation_4/1
  motorRotor4/3(torque) -> torque/1
  motorRotor4/1(thrust) -> thrust/1
  Signal_Saturation_4/1 -> Throttle To RPM Gain and Cutoff_8/1(In5)
  Df/1 -> motorRotor4/2(Df)
  Vs/1 -> Throttle To RPM Gain and Cutoff_8/2(Vs)

== system MavicProComplete/Quadcopter/Powertrain/motorGroup/motor4 ==
  note: Throttle cutoff can simulate the fact that the motor doesn't
      | spin until a minimum throttle point is reached. This introduces
      | a jump discontinuity in low throttle performance.
  note: These saturations model a SIGNAL LIMITATION.
      | Other intentional control saturations might be introduced in the
      | control loop to achieve better stability and consistency.
  throttleIn : Inport
  Df : Inport  Port=2
  Vs : Inport  Port=3
  Scope : Scope
  Signal_Saturation_4 : Saturate  UpperLimit=100  LowerLimit=0
  Throttle To RPM Gain and Cutoff_8 : Subsystem
  motorRotor4 : Subsystem
  thrust : Outport
  rpm : Outport  Port=2
  torque : Outport  Port=3
  current : Outport  Port=4
  wires:
  Throttle To RPM Gain and Cutoff_8/1(Out5) -> motorRotor4/1(V), Scope/1
  motorRotor4/4(current) -> current/1
  motorRotor4/2(rpm) -> rpm/1
  throttleIn/1 -> Signal_Saturation_4/1
  motorRotor4/3(torque) -> torque/1
  motorRotor4/1(thrust) -> thrust/1
  Signal_Saturation_4/1 -> Throttle To RPM Gain and Cutoff_8/1(In5)
  Df/1 -> motorRotor4/2(Df)
  Vs/1 -> Throttle To RPM Gain and Cutoff_8/2(Vs)

== system MavicProComplete/Quadcopter/Powertrain/motorGroup/motor1/Throttle To RPM Gain and Cutoff_8 ==
  note: Output equals linearly scaled RPM
      | for given throttle input if throttle input >=Throttle Cuttoff (minThr)
      | else output is zero.
  In5 : Inport
  Vs : Inport  Port=2
  Gain : Gain  Gain=.01
  Minimum Throttle Cutoff : simulink/Logic and Bit Operations/Compare To Constant  relop=>=  const=5  OutDataTypeStr=uint8
  Product : Product
  Product2 : Product
  Out5 : Outport
  wires:
  Minimum Throttle Cutoff/1 -> Product/2
  Product/1 -> Out5/1
  In5/1 -> Gain/1, Minimum Throttle Cutoff/1
  Gain/1 -> Product2/2
  Product2/1 -> Product/1
  Vs/1 -> Product2/1

== system MavicProComplete/Quadcopter/Powertrain/motorGroup/motor1/motorRotor4 ==
  V : Inport
  Df : Inport  Port=2
  Electrical part : Subsystem
  Mechanical part : Subsystem
  thrust : Outport
  rpm : Outport  Port=2
  torque : Outport  Port=3
  current : Outport  Port=4
  wires:
  V/1 -> Electrical part/1(Vin)
  Mechanical part/2(Thrust) -> thrust/1
  Electrical part/1(Electrical Torque) -> Mechanical part/2(Electrical Torque)
  Mechanical part/4(Torque) -> torque/1
  Mechanical part/1(w angular speed) -> Electrical part/2(w angular speed)
  Df/1 -> Mechanical part/1(dynamicFriction)
  Electrical part/2(current) -> current/1
  Mechanical part/3(rpm) -> rpm/1

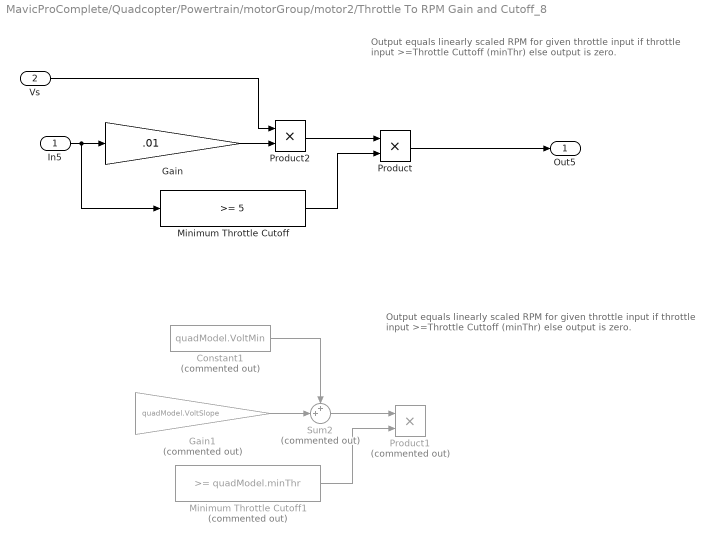
== system MavicProComplete/Quadcopter/Powertrain/motorGroup/motor2/Throttle To RPM Gain and Cutoff_8 ==
  note: Output equals linearly scaled RPM
      | for given throttle input if throttle input >=Throttle Cuttoff (minThr)
      | else output is zero.
  note: Output equals linearly scaled RPM
      | for given throttle input if throttle input >=Throttle Cuttoff (minThr)
      | else output is zero.
  In5 : Inport
  Vs : Inport  Port=2
  Constant1 : Constant  Commented=on  Value=quadModel.VoltMin
  Gain : Gain  Gain=.01
  Gain1 : Gain  Commented=on  Gain=quadModel.VoltSlope
  Minimum Throttle Cutoff : simulink/Logic and Bit Operations/Compare To Constant  relop=>=  const=5  OutDataTypeStr=uint8
  Minimum Throttle Cutoff1 : simulink/Logic and Bit Operations/Compare To Constant  Commented=on  relop=>=  const=quadModel.minThr  OutDataTypeStr=uint8
  Product : Product
  Product1 : Product  Commented=on
  Product2 : Product
  Sum2 : Sum  Commented=on  Inputs=++|
  Out5 : Outport
  wires:
  Minimum Throttle Cutoff/1 -> Product/2
  Product/1 -> Out5/1
  In5/1 -> Gain/1, Minimum Throttle Cutoff/1
  Gain/1 -> Product2/2
  Product2/1 -> Product/1
  Gain1/1 -> Sum2/2
  Constant1/1 -> Sum2/1
  Sum2/1 -> Product1/1
  Minimum Throttle Cutoff1/1 -> Product1/2
  Vs/1 -> Product2/1

== system MavicProComplete/Quadcopter/Powertrain/motorGroup/motor2/motorRotor4 ==
  V : Inport
  Df : Inport  Port=2
  Convert rad/s to rmp : Gain  Gain=60/(2*pi)
  Electrical part : Subsystem
  Mechanical part : Subsystem
  thrust : Outport
  rpm : Outport  Port=2
  torque : Outport  Port=3
  current : Outport  Port=4
  wires:
  Convert rad/s to rmp/1 -> rpm/1
  V/1 -> Electrical part/1(ESC voltage)
  Mechanical part/2(Thrust) -> thrust/1
  Electrical part/1(Electrical Torque) -> Mechanical part/2(Electrical Torque)
  Mechanical part/3(Torque) -> torque/1
  Mechanical part/1(w angular speed) -> Electrical part/2(w angular speed), Convert rad/s to rmp/1
  Df/1 -> Mechanical part/1(dynamicFriction)
  Electrical part/2(current) -> current/1

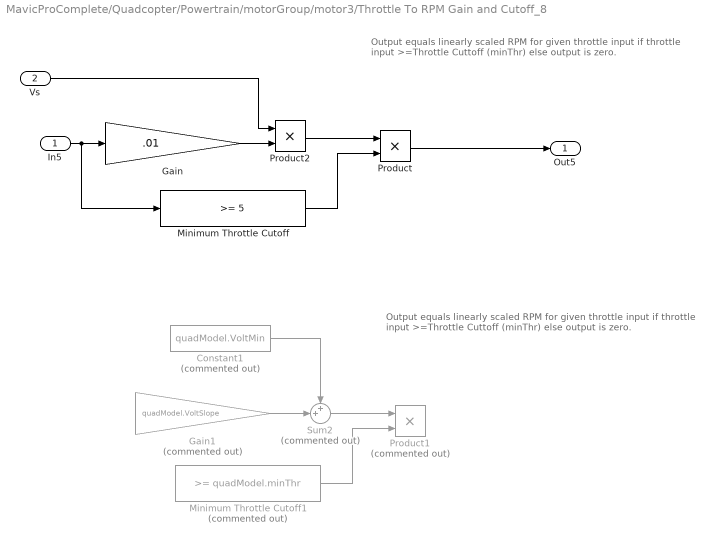
== system MavicProComplete/Quadcopter/Powertrain/motorGroup/motor3/Throttle To RPM Gain and Cutoff_8 ==
  note: Output equals linearly scaled RPM
      | for given throttle input if throttle input >=Throttle Cuttoff (minThr)
      | else output is zero.
  note: Output equals linearly scaled RPM
      | for given throttle input if throttle input >=Throttle Cuttoff (minThr)
      | else output is zero.
  In5 : Inport
  Vs : Inport  Port=2
  Constant1 : Constant  Commented=on  Value=quadModel.VoltMin
  Gain : Gain  Gain=.01
  Gain1 : Gain  Commented=on  Gain=quadModel.VoltSlope
  Minimum Throttle Cutoff : simulink/Logic and Bit Operations/Compare To Constant  relop=>=  const=5  OutDataTypeStr=uint8
  Minimum Throttle Cutoff1 : simulink/Logic and Bit Operations/Compare To Constant  Commented=on  relop=>=  const=quadModel.minThr  OutDataTypeStr=uint8
  Product : Product
  Product1 : Product  Commented=on
  Product2 : Product
  Sum2 : Sum  Commented=on  Inputs=++|
  Out5 : Outport
  wires:
  Minimum Throttle Cutoff/1 -> Product/2
  Product/1 -> Out5/1
  In5/1 -> Gain/1, Minimum Throttle Cutoff/1
  Gain/1 -> Product2/2
  Product2/1 -> Product/1
  Gain1/1 -> Sum2/2
  Constant1/1 -> Sum2/1
  Sum2/1 -> Product1/1
  Minimum Throttle Cutoff1/1 -> Product1/2
  Vs/1 -> Product2/1

== system MavicProComplete/Quadcopter/Powertrain/motorGroup/motor3/motorRotor4 ==
  V : Inport
  Df : Inport  Port=2
  Convert rad/s to rmp : Gain  Gain=60/(2*pi)
  Electrical part : Subsystem
  Mechanical part : Subsystem
  thrust : Outport
  rpm : Outport  Port=2
  torque : Outport  Port=3
  current : Outport  Port=4
  wires:
  Convert rad/s to rmp/1 -> rpm/1
  V/1 -> Electrical part/1(ESC voltage)
  Mechanical part/2(Thrust) -> thrust/1
  Electrical part/1(Electrical Torque) -> Mechanical part/2(Electrical Torque)
  Mechanical part/3(Torque) -> torque/1
  Mechanical part/1(w angular speed) -> Electrical part/2(w angular speed), Convert rad/s to rmp/1
  Df/1 -> Mechanical part/1(dynamicFriction)
  Electrical part/2(current) -> current/1

== system MavicProComplete/Quadcopter/Powertrain/motorGroup/motor4/Throttle To RPM Gain and Cutoff_8 ==
  note: Output equals linearly scaled RPM
      | for given throttle input if throttle input >=Throttle Cuttoff (minThr)
      | else output is zero.
  note: Output equals linearly scaled RPM
      | for given throttle input if throttle input >=Throttle Cuttoff (minThr)
      | else output is zero.
  In5 : Inport
  Vs : Inport  Port=2
  Constant1 : Constant  Commented=on  Value=quadModel.VoltMin
  Gain : Gain  Gain=.01
  Gain1 : Gain  Commented=on  Gain=quadModel.VoltSlope
  Minimum Throttle Cutoff : simulink/Logic and Bit Operations/Compare To Constant  relop=>=  const=5  OutDataTypeStr=uint8
  Minimum Throttle Cutoff1 : simulink/Logic and Bit Operations/Compare To Constant  Commented=on  relop=>=  const=quadModel.minThr  OutDataTypeStr=uint8
  Product : Product
  Product1 : Product  Commented=on
  Product2 : Product
  Sum2 : Sum  Commented=on  Inputs=++|
  Out5 : Outport
  wires:
  Minimum Throttle Cutoff/1 -> Product/2
  Product/1 -> Out5/1
  In5/1 -> Gain/1, Minimum Throttle Cutoff/1
  Gain/1 -> Product2/2
  Product2/1 -> Product/1
  Gain1/1 -> Sum2/2
  Constant1/1 -> Sum2/1
  Sum2/1 -> Product1/1
  Minimum Throttle Cutoff1/1 -> Product1/2
  Vs/1 -> Product2/1

== system MavicProComplete/Quadcopter/Powertrain/motorGroup/motor4/motorRotor4 ==
  V : Inport
  Df : Inport  Port=2
  Convert rad/s to rmp : Gain  Gain=60/(2*pi)
  Electrical part : Subsystem
  Mechanical part : Subsystem
  thrust : Outport
  rpm : Outport  Port=2
  torque : Outport  Port=3
  current : Outport  Port=4
  wires:
  Convert rad/s to rmp/1 -> rpm/1
  V/1 -> Electrical part/1(ESC voltage)
  Mechanical part/2(Thrust) -> thrust/1
  Electrical part/1(Electrical Torque) -> Mechanical part/2(Electrical Torque)
  Mechanical part/3(Torque) -> torque/1
  Mechanical part/1(w angular speed) -> Electrical part/2(w angular speed), Convert rad/s to rmp/1
  Df/1 -> Mechanical part/1(dynamicFriction)
  Electrical part/2(current) -> current/1

== system MavicProComplete/Quadcopter/Powertrain/motorGroup/motor1/motorRotor4/Electrical part ==
  Vin : Inport
  w angular speed : Inport  Port=2
  1/R : Gain  Gain=1/Motor.Req
  Ke (Torque constant)1 : Gain  Gain=Motor.Ke_eq
  Kt (Torque constant) Kt=Ke for an ideal square wave motor : Gain  Gain=Motor.Ke_eq
  Sum : Sum  Inputs=|+-
  Electrical Torque : Outport
  current : Outport  Port=2
  wires:
  1/R/1 -> current/1, Kt (Torque constant) Kt=Ke for an ideal square wave motor/1  "current i"
  Sum/1 -> 1/R/1
  Kt (Torque constant) Kt=Ke for an ideal square wave motor/1 -> Electrical Torque/1
  Ke (Torque constant)1/1 -> Sum/2
  Vin/1 -> Sum/1
  w angular speed/1 -> Ke (Torque constant)1/1

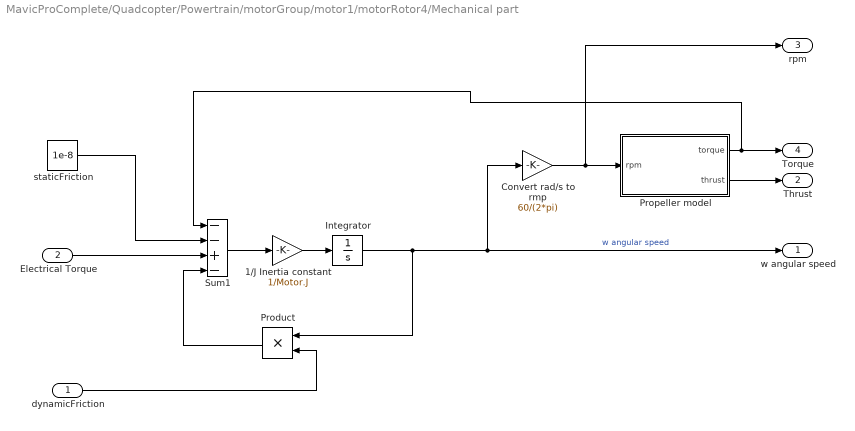
== system MavicProComplete/Quadcopter/Powertrain/motorGroup/motor1/motorRotor4/Mechanical part ==
  dynamicFriction : Inport
  Electrical Torque : Inport  Port=2
  1/J Inertia constant : Gain  Gain=1/Motor.J
  Convert rad/s to rmp : Gain  Gain=60/(2*pi)
  Integrator : Integrator  InitialCondition=419
  Product : Product
  "Propeller model " : MATLAB Function  TreatAsAtomicUnit=on
  Sum1 : Sum  Inputs=--+-
  staticFriction : Constant  Value=1e-8
  w angular speed : Outport
  Thrust : Outport  Port=2
  rpm : Outport  Port=3
  Torque : Outport  Port=4
  wires:
  "Propeller model "/1(torque) -> Sum1/1, Torque/1
  1/J Inertia constant/1 -> Integrator/1
  dynamicFriction/1 -> Product/2
  Product/1 -> Sum1/4
  Integrator/1 -> Product/1, w angular speed/1, Convert rad/s to rmp/1  "w angular speed"
  Sum1/1 -> 1/J Inertia constant/1
  Electrical Torque/1 -> Sum1/3
  Convert rad/s to rmp/1 -> rpm/1, "Propeller model "/1(rpm)
  "Propeller model "/2(thrust) -> Thrust/1
  staticFriction/1 -> Sum1/2

== system MavicProComplete/Quadcopter/Powertrain/motorGroup/motor2/motorRotor4/Electrical part ==
  ESC voltage : Inport
  w angular speed : Inport  Port=2
  1/R : Gain  Gain=1/Motor.Req
  Ke (Torque constant)1 : Gain  Gain=Motor.Ke_eq
  Kt (Torque constant) Kt=Ke for an ideal square wave motor : Gain  Gain=Motor.Ke_eq
  Sum : Sum  Inputs=|+-
  Electrical Torque : Outport
  current : Outport  Port=2
  wires:
  1/R/1 -> current/1, Kt (Torque constant) Kt=Ke for an ideal square wave motor/1  "current i"
  Sum/1 -> 1/R/1
  Kt (Torque constant) Kt=Ke for an ideal square wave motor/1 -> Electrical Torque/1
  Ke (Torque constant)1/1 -> Sum/2
  ESC voltage/1 -> Sum/1
  w angular speed/1 -> Ke (Torque constant)1/1

== system MavicProComplete/Quadcopter/Powertrain/motorGroup/motor2/motorRotor4/Mechanical part ==
  dynamicFriction : Inport
  Electrical Torque : Inport  Port=2
  1/J Inertia constant : Gain  Gain=1/Motor.J
  Convert rad/s to rmp : Gain  Gain=60/(2*pi)
  Integrator : Integrator  InitialCondition=419
  Product : Product
  "Propeller model " : MATLAB Function  TreatAsAtomicUnit=on
  Sum1 : Sum  Inputs=--+-
  staticFriction : Constant  Value=1e-8
  w angular speed : Outport
  Thrust : Outport  Port=2
  Torque : Outport  Port=3
  wires:
  "Propeller model "/1(torque) -> Sum1/1, Torque/1
  1/J Inertia constant/1 -> Integrator/1
  dynamicFriction/1 -> Product/2
  Product/1 -> Sum1/4
  Integrator/1 -> Product/1, w angular speed/1, Convert rad/s to rmp/1  "w angular speed"
  Sum1/1 -> 1/J Inertia constant/1
  Electrical Torque/1 -> Sum1/3
  Convert rad/s to rmp/1 -> "Propeller model "/1(rpm)
  "Propeller model "/2(thrust) -> Thrust/1
  staticFriction/1 -> Sum1/2

== system MavicProComplete/Quadcopter/Powertrain/motorGroup/motor3/motorRotor4/Electrical part ==
  ESC voltage : Inport
  w angular speed : Inport  Port=2
  1/R : Gain  Gain=1/Motor.Req
  Ke (Torque constant)1 : Gain  Gain=Motor.Ke_eq
  Kt (Torque constant) Kt=Ke for an ideal square wave motor : Gain  Gain=Motor.Ke_eq
  Sum : Sum  Inputs=|+-
  Electrical Torque : Outport
  current : Outport  Port=2
  wires:
  1/R/1 -> current/1, Kt (Torque constant) Kt=Ke for an ideal square wave motor/1  "current i"
  Sum/1 -> 1/R/1
  Kt (Torque constant) Kt=Ke for an ideal square wave motor/1 -> Electrical Torque/1
  Ke (Torque constant)1/1 -> Sum/2
  ESC voltage/1 -> Sum/1
  w angular speed/1 -> Ke (Torque constant)1/1

== system MavicProComplete/Quadcopter/Powertrain/motorGroup/motor3/motorRotor4/Mechanical part ==
  dynamicFriction : Inport
  Electrical Torque : Inport  Port=2
  1/J Inertia constant : Gain  Gain=1/Motor.J
  Convert rad/s to rmp : Gain  Gain=60/(2*pi)
  Integrator : Integrator  InitialCondition=419
  Product : Product
  "Propeller model " : MATLAB Function  TreatAsAtomicUnit=on
  Sum1 : Sum  Inputs=--+-
  staticFriction : Constant  Value=1e-8
  w angular speed : Outport
  Thrust : Outport  Port=2
  Torque : Outport  Port=3
  wires:
  "Propeller model "/1(torque) -> Sum1/1, Torque/1
  1/J Inertia constant/1 -> Integrator/1
  dynamicFriction/1 -> Product/2
  Product/1 -> Sum1/4
  Integrator/1 -> Product/1, w angular speed/1, Convert rad/s to rmp/1  "w angular speed"
  Sum1/1 -> 1/J Inertia constant/1
  Electrical Torque/1 -> Sum1/3
  Convert rad/s to rmp/1 -> "Propeller model "/1(rpm)
  "Propeller model "/2(thrust) -> Thrust/1
  staticFriction/1 -> Sum1/2

== system MavicProComplete/Quadcopter/Powertrain/motorGroup/motor4/motorRotor4/Electrical part ==
  ESC voltage : Inport
  w angular speed : Inport  Port=2
  1/R : Gain  Gain=1/Motor.Req
  Ke (Torque constant)1 : Gain  Gain=Motor.Ke_eq
  Kt (Torque constant) Kt=Ke for an ideal square wave motor : Gain  Gain=Motor.Ke_eq
  Sum : Sum  Inputs=|+-
  Electrical Torque : Outport
  current : Outport  Port=2
  wires:
  1/R/1 -> current/1, Kt (Torque constant) Kt=Ke for an ideal square wave motor/1  "current i"
  Sum/1 -> 1/R/1
  Kt (Torque constant) Kt=Ke for an ideal square wave motor/1 -> Electrical Torque/1
  Ke (Torque constant)1/1 -> Sum/2
  ESC voltage/1 -> Sum/1
  w angular speed/1 -> Ke (Torque constant)1/1

== system MavicProComplete/Quadcopter/Powertrain/motorGroup/motor4/motorRotor4/Mechanical part ==
  dynamicFriction : Inport
  Electrical Torque : Inport  Port=2
  1/J Inertia constant : Gain  Gain=1/Motor.J
  Convert rad/s to rmp : Gain  Gain=60/(2*pi)
  Integrator : Integrator  InitialCondition=419
  Product : Product
  "Propeller model " : MATLAB Function  TreatAsAtomicUnit=on
  Sum1 : Sum  Inputs=--+-
  staticFriction : Constant  Value=1e-8
  w angular speed : Outport
  Thrust : Outport  Port=2
  Torque : Outport  Port=3
  wires:
  "Propeller model "/1(torque) -> Sum1/1, Torque/1
  1/J Inertia constant/1 -> Integrator/1
  dynamicFriction/1 -> Product/2
  Product/1 -> Sum1/4
  Integrator/1 -> Product/1, w angular speed/1, Convert rad/s to rmp/1  "w angular speed"
  Sum1/1 -> 1/J Inertia constant/1
  Electrical Torque/1 -> Sum1/3
  Convert rad/s to rmp/1 -> "Propeller model "/1(rpm)
  "Propeller model "/2(thrust) -> Thrust/1
  staticFriction/1 -> Sum1/2

== matlab function MavicProComplete/Quadcopter/Powertrain/motorGroup/motor1/motorRotor4/Mechanical part/Propeller model  ==
  data: torque output; rpm input; thrust output
function [torque,thrust] = fcn(rpm)
% angular_velocity in rpm

%coefficient of thrust, empirically derived
coef_t = 2*(10^-15)*rpm^3 - 4*(10^-11)*rpm^2 + 3*(10^-7)*rpm + .1013;
%thrust = coef_t * density of air * velocity^2 * propeller diameter (m) ^4
thrust = coef_t*1.225*(rpm/60)^2*.2^4;
% empirically derived
torque = 4*(10^-14)*rpm^3 +  8*(10^-12)*rpm^2 + 3*(10^-6)*rpm;
end

== matlab function MavicProComplete/Quadcopter/Powertrain/motorGroup/motor2/motorRotor4/Mechanical part/Propeller model  ==
  data: torque output; rpm input; thrust output
function [torque,thrust] = fcn(rpm)
% angular_velocity in rpm

%coefficient of thrust, empirically derived
coef_t = 2*(10^-15)*rpm^3 - 4*(10^-11)*rpm^2 + 3*(10^-7)*rpm + .1013;
%thrust = coef_t * density of air * velocity^2 * propeller diameter (m) ^4
thrust = coef_t*1.225*(rpm/60)^2*.2^4;
% empirically derived
torque = 4*(10^-14)*rpm^3 +  8*(10^-12)*rpm^2 + 3*(10^-6)*rpm;
end

== matlab function MavicProComplete/Quadcopter/Powertrain/motorGroup/motor3/motorRotor4/Mechanical part/Propeller model  ==
  data: torque output; rpm input; thrust output
function [torque,thrust] = fcn(rpm)
% angular_velocity in rpm

%coefficient of thrust, empirically derived
coef_t = 2*(10^-15)*rpm^3 - 4*(10^-11)*rpm^2 + 3*(10^-7)*rpm + .1013;
%thrust = coef_t * density of air * velocity^2 * propeller diameter (m) ^4
thrust = coef_t*1.225*(rpm/60)^2*.2^4;
% empirically derived
torque = 4*(10^-14)*rpm^3 +  8*(10^-12)*rpm^2 + 3*(10^-6)*rpm;
end
